simulink model "Contoller"  (R2019a)
settings: Solver=FixedStepDiscrete  StartTime=0.0  StopTime=40  FixedStep=0.25  RelTol=1e-3
settings Model: Creator=Athar Hussain  LastModifiedBy=Athar Hussain

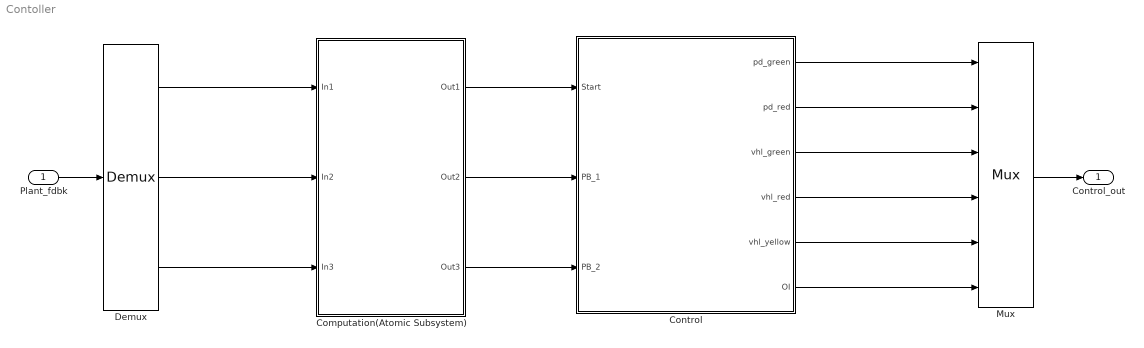
== system Contoller ==
  Plant_fdbk : Inport
  Computation(Atomic Subsystem) : Subsystem  TreatAsAtomicUnit=on
  Control : Stateflow chart  BlockKeywords=__PRM__SERIALIZED__DATA__:Stateflow Chart,Stateflow Diagram  TreatAsAtomicUnit=on
  Demux : Demux  Outputs=3
  Mux : Mux  Inputs=6
  Control_out : Outport
  wires:
  Mux/1 -> Control_out/1
  Plant_fdbk/1 -> Demux/1
  Control/1(pd_green) -> Mux/1
  Control/2(pd_red) -> Mux/2
  Control/3(vhl_green) -> Mux/3
  Control/4(vhl_red) -> Mux/4
  Control/5(vhl_yellow) -> Mux/5
  Control/6(OI) -> Mux/6
  Demux/1 -> Computation(Atomic Subsystem)/1(In1)
  Demux/2 -> Computation(Atomic Subsystem)/2(In2)
  Demux/3 -> Computation(Atomic Subsystem)/3(In3)
  Computation(Atomic Subsystem)/1(Out1) -> Control/1(Start)
  Computation(Atomic Subsystem)/2(Out2) -> Control/2(PB_1)
  Computation(Atomic Subsystem)/3(Out3) -> Control/3(PB_2)

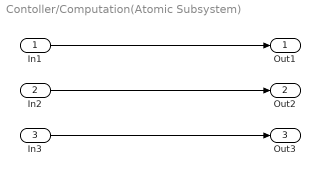
== system Contoller/Computation(Atomic Subsystem) ==
  In1 : Inport
  In2 : Inport  Port=2
  In3 : Inport  Port=3
  Out1 : Outport
  Out2 : Outport  Port=2
  Out3 : Outport  Port=3
  wires:
  In1/1 -> Out1/1
  In3/1 -> Out3/1
  In2/1 -> Out2/1

== stateflow chart Contoller/Control ==
  settings: executeAtInitialization=1
  state Intit
    entry:
    x = 0;
    wait_cross = 20;
    vhl_green = 1;
    vhl_yellow = 1;
    vhl_red = 1;
    pd_green = 0;
    pd_red = 0;
    OI = 0;
  state [WAIT_CROSS,oi] = check_PB(pb_1, pb_2) [function]
    (default) -> (junction 159) : {WAIT_CROSS=20;oi=0;}% check_PB
    (junction 159) -> (junction 160) [order 1] : [(x == 0 & pb_1 == 1 | pb_2 == 1)]
    (junction 159) -> (junction 161) [order 2]
    (junction 160) -> (junction 165) : {WAIT_CROSS = 15; oi = 1; x=1;}
    (junction 161) -> (junction 162) [order 1] : [x == 1]
    (junction 161) -> (junction 163) [order 2]
    (junction 162) -> (junction 164) : {WAIT_CROSS = 15; oi = 1;}
    (junction 164) -> (junction 163)
    (junction 165) -> (junction 164)
    (junction 163) -> (junction 166)
  state vhl_stopp
    entry:
    vhl_green = 0;
    vhl_yellow = 0;
    vhl_red = 1;
    pd_green = 1;
    pd_red = 0;
    OI = 0;
  state vhl_pre_stopp
    entry:
    vhl_green = 0;
    vhl_yellow = 1;
    vhl_red = 0;
    pd_green = 0;
    pd_red =1;
    during:
    [wait_cross,OI] = check_PB(PB_1,PB_2);
  state vhl_pre_cross
    entry:
    vhl_green = 0;
    vhl_yellow = 1;
    vhl_red = 1;
    pd_green = 0;
    pd_red = 1;
    during:
    [wait_cross, OI] = check_PB(PB_1,PB_2);
  state vlh_cross
    entry:
    vhl_green = 1;
    vhl_yellow = 0;
    vhl_red = 0;
    pd_green = 0;
    pd_red = 1;
    during:
    [wait_cross,OI] = check_PB(PB_1,PB_2);
  (default) -> Intit
  vhl_pre_stopp -> Intit [order 1] : [Start == 0]
  Intit -> vhl_stopp : [Start == 1]
  vhl_pre_stopp -> vhl_stopp [order 2] : after(3,sec){x = 0;}
  vhl_stopp -> vhl_pre_cross : after(10,sec)
  vlh_cross -> vhl_pre_stopp : after(wait_cross,sec)
  vhl_pre_cross -> vlh_cross : after(5,sec)
  data: pb_1 function_input; pb_2 function_input; WAIT_CROSS function_output; oi function_output; Start input; PB_1 input; PB_2 input; pd_green output; pd_red output; vhl_green output; vhl_red output; vhl_yellow output; wait_cross local =20; OI output; x local =0
